simulink model "model_3dof_steering_lateral_selfmade"  (R2022a)
settings: Solver=ode15s  StartTime=0.0  StopTime=para_dura  FixedStep=para_sim_step  MaxStep=para_sim_step  RelTol=1e-9
model workspace (MAT data in the model file):
  SCD_FRESTIMATE_Operating_Point = opcond.OperatingPoint
  SCD_FRESTIMATE_Operating_Point.Model_ = 'model_1dof_longitudinal'
  SCD_FRESTIMATE_Operating_Point.States_(1) = opcond.StatePoint
  SCD_FRESTIMATE_Operating_Point.States_(1).Nx_ = 41
  SCD_FRESTIMATE_Operating_Point.States_(1).Block_ = 'model_1dof_longitudinal/Excitation System/Int Operator'
  SCD_FRESTIMATE_Operating_Point.States_(1).StateName_ = 'v'
  SCD_FRESTIMATE_Operating_Point.States_(1).x_ = [2.02683501926e-10; 1.37568821264e-19; 7.14890844399e-22; 1.12455204277e-20; -7.0630005675e-20; -6.95938068614e-20; 2.72721447959e-21; -3.93535312325e-20; -1.14815977745e-19; 3.30570889294e-20; 3.78600196645e-20; 7.21851569254e-20; -1.77555585105e-19; -2.35291525241e-20; 4.41713994739e-20; -2.05900764101e-21; -1.58367864176e-20; 6.35039836383e-20; -1.30347120926e-20; 1.28680290784e-21; 5.17371795703e-20; 6.49899736287e-20; -4.65181773693e-21; 5.74556218522e-21; -3.90326541642e-20; -4.95314223748e-20; -4.80167923753e-19; 9.22449192438e-20; -2.20085792962e-21; -4.30092800651e-20; -3.42774380714e-20; -1.20947897418e-20; -3.0642370533e-20; -6.43164282462e-20; -2.97515387843e-19; -1.68698506591e-20; 2.312266433e-19; -7.84373380068e-21; 1.67577252929e-20; 2.59801809162e-21; -7.43993193604e-23]
  SCD_FRESTIMATE_Operating_Point.States_(2) = opcond.StatePoint
  SCD_FRESTIMATE_Operating_Point.States_(2).Nx_ = 1
  SCD_FRESTIMATE_Operating_Point.States_(2).Block_ = 'model_1dof_longitudinal/Vehicle Body 1DOF Longitudinal/Vehicle Body 1 DOF/Bus Creation/Body Frame/Longitudinal 1DOF/Integrator3'
  SCD_FRESTIMATE_Operating_Point.States_(2).x_ = 7.28555022085e-16
  SCD_FRESTIMATE_Operating_Point.States_(3) = opcond.StatePoint
  SCD_FRESTIMATE_Operating_Point.States_(3).Nx_ = 1
  SCD_FRESTIMATE_Operating_Point.States_(3).Block_ = 'model_1dof_longitudinal/Vehicle Body 1DOF Longitudinal/Vehicle Body 1 DOF/Integrator1'
  SCD_FRESTIMATE_Operating_Point.States_(3).x_ = -8.63730588445e-16
  SCD_FRESTIMATE_Operating_Point.States_(4) = opcond.StatePoint
  SCD_FRESTIMATE_Operating_Point.States_(4).Nx_ = 1
  SCD_FRESTIMATE_Operating_Point.States_(4).Block_ = 'model_1dof_longitudinal/Vehicle Body 1DOF Longitudinal/Vehicle Body 1 DOF/Vehicle/Integrator'
  SCD_FRESTIMATE_Operating_Point.States_(4).x_ = 1.82750662194e-20
values from neighbouring files (symbols this model uses):
  para_mats = paraStruct.Sv    [main_lateral.m]    (also in main_steering_lateral.m)
  para_sim_matu = paraStruct.SimUv    [main_lateral.m]    (also in main_steering_lateral.m)
  para_sim_step = 5e-4/2    (= 0.00025)    [main_lateral.m]    (also in main_steering_lateral.m = 0.005)
  para_vinit = paraStruct.VInit    [main_lateral.m]    (also in main_steering_lateral.m)
  sim_iun = Simulink.Parameter(1)    [main_lateral.m]    (also in main_steering_lateral.m)
  sim_usnr = zeros(para_sim_usize, 1)    [main_lateral.m]    (also in main_steering_lateral.m)
  ut_pwr = genPower(sim_ut, para_sim_usize)    [main_lateral.m]    (also in main_steering_lateral.m)
undefined symbols (not defined in the file or in its folder): AngSft, AngSW, AVelSft, AVelSW, dpsi, dy, fyf, fyr
libraries: simulink x1
settings Model: SimulationMode=accelerator  PacingRate=1.100000  Creator=无垠穹宇  LastModifiedBy=无垠穹宇
settings SolverCC: ZeroCrossAlgorithm=Adaptive  SolverResetMethod=Robust  MinimalZcImpactIntegration=on  EnableFixedStepZeroCrossing=on
settings DataIOCC: SaveOutput=off  SignalLogging=off  DSMLogging=off  SignalLoggingName=yt
settings OptimizationCC: DefaultParameterBehavior=Inlined  GainParamInheritBuiltInType=on  UseFloatMulNetSlope=on  InlineInvariantSignals=on  EnhancedBackFolding=on  PassReuseOutputArgsThreshold=0  EfficientFloat2IntCast=on  SimCompilerOptimization=on  OptimizeBlockOrder=speed  DifferentSizesBufferReuse=on
settings DebuggingCC: ReadBeforeWriteMsg=DisableAll  WriteAfterWriteMsg=DisableAll  WriteAfterReadMsg=DisableAll  IgnoredZcDiagnostic=none  SolverPrmCheckMsg=warning  MultiTaskDSMMsg=none  ParameterTunabilityLossMsg=error  StateNameClashWarn=warning
settings ModelReferenceCC: UpdateModelReferenceTargets=IfOutOfDate
settings SFSimCC: SFSimEcho=off  SimHardwareAcceleration=native
settings RTWCC: Description=Generic Real-Time Target  RetainRTWFile=on  BuildConfiguration=Faster Runs  CheckMdlBeforeBuild=Warning  DLArmComputeVersion=19.05
settings CodeAppCC: ForceParamTrailComments=on  OperatorAnnotations=on
settings GRTTargetCC: MatFileLogging=off  SupportNonFinite=off

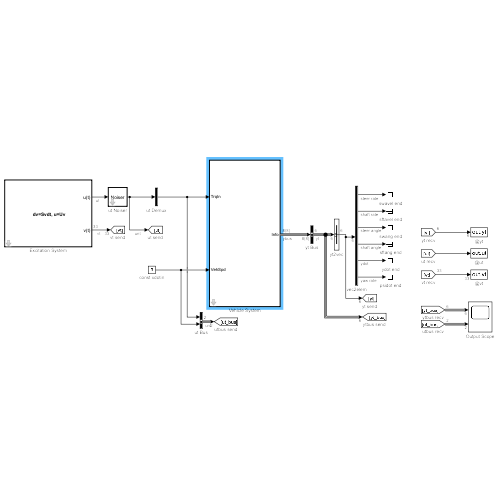
[thumbnail: Simulink's stored preview of the top-level diagram]
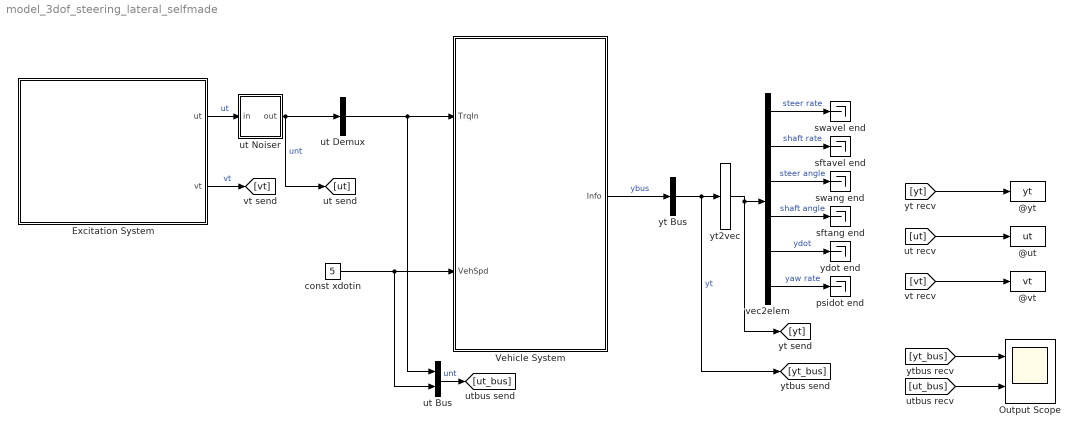
== system model_3dof_steering_lateral_selfmade ==
  @ut : ToWorkspace  VariableName=ut  SaveFormat=Timeseries  SampleTime=para_sim_step
      settings: Decimation=para_resamples
  @vt : ToWorkspace  VariableName=vt  SaveFormat=Timeseries  SampleTime=para_sim_step
      settings: Decimation=para_resamples
  @yt : ToWorkspace  VariableName=yt  SaveFormat=Timeseries  SampleTime=para_sim_step
      settings: Decimation=para_resamples
  Excitation System : Subsystem  TreatAsAtomicUnit=on  mask(State Space with State Vector Output){S=para_mats, U=para_sim_matu, v0=para_vinit}
      mask prompts: S "Matrix S"; U "Matrix U"; v0 "v(0)"
      mask help: 带状态输出的状态空间模型(无控制输入)
      mask DialogControl ParameterGroupVar Prompt: 参数
      mask Display:
      | disp('\bf dv=Svdt, u=Uv', 'texmode', 'on');
      | port_label('output', 1, 'u(t)');
      | port_label('output', 2, 'v(t)');
  Output Scope : Scope  NumInputPorts=2
  Vehicle System : Subsystem  TreatAsAtomicUnit=on  mask(Math Model Parameters){wCf=12e3, wCr=11e3, wIzz=4000, wJ1=0.1, wJ2=0.01, wK=30, wb1=0.001, wb2=1, wb3=0.001, wlf=1.4, wlr=1.6, wm=2000, wxi=0.3, wh=0.35, wTW=1.4, wFznom=5000, wg=9.81}
      mask prompts: wCf "Cf"; wCr "Cr"; wIzz "Izz"; wJ1 "J1"; wJ2 "J2"; wK "K"; wb1 "b1"; wb2 "b2"; wb3 "b3"; wlf "lf"; wlr "lr"; wm "m"; wxi "xi"; wh "h"; wTW "TW"; wFznom "Fznom"; wg "g"
      mask help: 输入状态方程参数, 国际单位制
      settings: MinAlgLoopOccurrences=on
      mask DialogControl ParameterGroupVar Prompt: 参数
  const xdotin : Constant  Value=5  VectorParams1D=off  OutDataTypeStr=double
  psidot end : Terminator
  sftang end : Terminator
  sftavel end : Terminator
  swang end : Terminator
  swavel end : Terminator
  ut Bus : BusCreator  Inputs=2
  ut Demux : Demux  Outputs=1
  ut Noiser : Subsystem  TreatAsAtomicUnit=on  mask(Vectorized AWGN){pwr=ut_pwr, snr=sim_usnr, fmax=20*para_sim_step, judge_para=sim_iun}
      mask prompts: pwr "信号功率向量 (W)"; snr "信噪比向量   (dB)"; fmax "最大动态频率 (1/rad)"; judge_para "噪声启用判断"
      mask help: 给定信号功率和信噪比, 添加高斯白噪声到信号中
      mask DialogControl ParameterGroupVar Prompt: 参数
      mask Display: disp('Noiser');
  vec2elem : Demux  Outputs=6
  ydot end : Terminator
  yt Bus : BusSelector  OutputSignals=shaft info.AVelSW,shaft info.AVelSft,shaft info.AngSW,shaft info.AngSft,body info.dy,body info.dpsi  OutputAsBus=on
  yt2vec : BusToVector
  wires:
  ut Bus/1 -> [ut_bus]  "unt"
  const xdotin/1 -> ut Bus/2, Vehicle System/2(VehSpd)
  ut Noiser/1(out) -> [ut], ut Demux/1  "unt"
  Excitation System/2(vt) -> [vt]  "vt"
  Excitation System/1(ut) -> ut Noiser/1(in)  "ut"
  vec2elem/6 -> psidot end/1  "yaw rate"
  vec2elem/4 -> sftang end/1  "shaft angle"
  vec2elem/5 -> ydot end/1  "ydot"
  yt2vec/1 -> [yt], vec2elem/1
  [yt] -> @yt/1
  vec2elem/3 -> swang end/1  "steer angle"
  [ut] -> @ut/1
  [ut_bus] -> Output Scope/2
  [yt_bus] -> Output Scope/1
  yt Bus/1 -> yt2vec/1, [yt_bus]  "yt"
  [vt] -> @vt/1
  vec2elem/2 -> sftavel end/1  "shaft rate"
  vec2elem/1 -> swavel end/1  "steer rate"
  Vehicle System/1(Info) -> yt Bus/1  "ybus"
  ut Demux/1 -> ut Bus/1, Vehicle System/1(TrqIn)

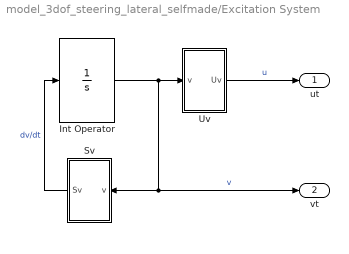
== system model_3dof_steering_lateral_selfmade/Excitation System ==
  Int Operator : Integrator  InitialCondition=v0  WrappedStateUpperValue=1  WrappedStateLowerValue=-1  ContinuousStateAttributes='v'
  Sv : Subsystem
      mask Display: disp('Sv');
  Uv : Subsystem
      mask Display: disp('Uv');
  ut : Outport  OutDataTypeStr=double
  vt : Outport  Port=2  OutDataTypeStr=double
  wires:
  Uv/1(Uv) -> ut/1  "u"
  Int Operator/1 -> Uv/1(v), vt/1, Sv/1(v)  "v"
  Sv/1(Sv) -> Int Operator/1  "dv/dt"

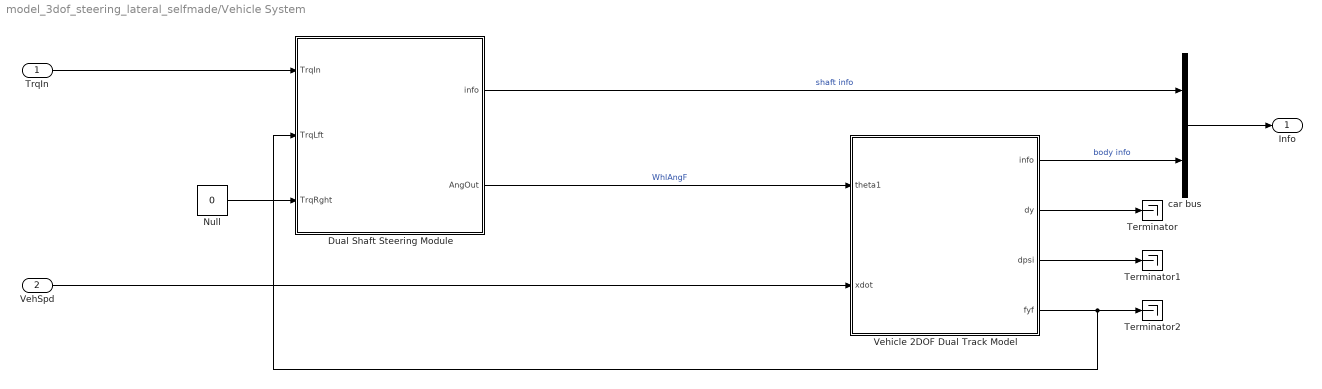
== system model_3dof_steering_lateral_selfmade/Vehicle System ==
  TrqIn : Inport
  VehSpd : Inport  Port=2
  Dual Shaft Steering Module : Subsystem  mask(Dual Shaft Dynamics){J1=wJ1, J2=wJ2, b1=wb1, k1=wK, b2=wb2, b3=wb3, theta_o=0, omega_o=0, xi=wxi, FricTrq=0}
      mask prompts: J1 "vdynblks:vehdynDynamicSteering:blkPrm_J1"; J2 "vdynblks:vehdynDynamicSteering:blkPrm_J2"; b1 "vdynblks:vehdynDynamicSteering:blkPrm_b1"; k1 "vdynblks:vehdynDynamicSteering:blkPrm_k1"; b2 "vdynblks:vehdynDynamicSteering:blkPrm_b3"; b3 "vdynblks:vehdynDynamicSteering:blkPrm_b2"; theta_o "vdynblks:vehdynDynamicSteering:blkPrm_theta_o"; omega_o "vdynblks:vehdynDynamicSteering:blkPrm_omega_o"; xi "trail + pneumatic trail (m)"; FricTrq "vdynblks:vehdynDynamicSteering:blkPrm_FricTrq"
      mask help: 见说明文档
      settings: MinAlgLoopOccurrences=on
      mask Help: eval('vdynblkshelp(''vbsteerdyn'')')
      mask DialogControl J1 Prompt: Steering wheel inertia, J1 [kg*m^2]:
      mask DialogControl J2 Prompt: Steering mechanism inertia, J2 [kg*m^2]:
      mask DialogControl b1 Prompt: Hysteresis viscous damping, b1 [N*m*s/rad]:
      mask DialogControl k1 Prompt: Hysteresis stiffness, k1 [N*m/rad]:
      mask DialogControl b2 Prompt: Steering wheel damping, b2 [N*m*s/rad]:
      mask DialogControl b3 Prompt: Steering mechanism damping, b3 [N*m*s/rad]:
      mask DialogControl theta_o Prompt: Initial steering angle, theta_o [rad]:
      mask DialogControl omega_o Prompt: Initial steering angular velocity, omega_o [rad/s]:
      mask DialogControl FricTrq Prompt: Friction torque, FricTrq [N*m]:
      mask Display:
      | disp('Dual Shaft Dynamics');
      | port_label('input', 1, 'TrqIn');
      | port_label('input', 2, 'TrqLft');
      | port_label('input', 3, 'TrqRght');
      | port_label('output', 1, 'info');
      | port_label('output', 2, 'AngOut');
  Null : Constant  Value=0
  Terminator : Terminator
  Terminator1 : Terminator
  Terminator2 : Terminator
  Vehicle 2DOF Dual Track Model : Subsystem  mask(Vehicle Body 3DOF Lateral){m=wm, h=wh, a=wlf, b=wlr, w=wTW, Cy_f=wCf, Cy_r=wCr, Izz=wIzz, Fznom=wm*wg, g=wg}
      mask prompts: m "autoblks_shared:autoblkVehBody3DofLat:blkPrm_m"; h "Vertical distance from center of mass to axle plane, h [m]:"; a "autoblks_shared:autoblkVehBody3DofLat:blkPrm_a"; b "autoblks_shared:autoblkVehBody3DofLat:blkPrm_b"; w "autoblks_shared:autoblkVehBody3DofLat:blkPrm_w"; Cy_f "autoblks_shared:autoblkVehBody3DofLat:blkPrm_Cy_f"; Cy_r "autoblks_shared:autoblkVehBody3DofLat:blkPrm_Cy_r"; Izz "autoblks_shared:autoblkVehBody3DofLat:blkPrm_Izz"; Fznom "autoblks_shared:autoblkVehBody3DofLat:blkPrm_Fznom"; g "Gravitational acceleration, g [m/s^2]:"
      mask help: autoblks_shared:autoblkVehBody3DofLat:blkDesc
      settings: MinAlgLoopOccurrences=on
      mask Help: eval('autosharedhelp(''vb3doflat'')');
      mask DialogControl ParameterGroupVar Prompt: autoblks_shared:autoblkVehBody3DofLat:blkDlg_ParameterGroupVar
      mask DialogControl LongPanel Prompt: autoblks_shared:autoblkVehBody3DofLat:blkDlg_LongPanel
      mask DialogControl m Prompt: Vehicle mass, m [kg]:
      mask DialogControl a Prompt: Longitudinal distance from center of mass to front axle, a [m]:
      mask DialogControl b Prompt: Longitudinal distance from center of mass to rear axle, b [m]:
      mask DialogControl LatPanel Prompt: autoblks_shared:autoblkVehBody3DofLat:blkDlg_LatPanel
      mask DialogControl w Prompt: Track width, w [m]:
      mask DialogControl Cy_f Prompt: Front tire corner stiffness, Cy_f [N/rad]:
      mask DialogControl Cy_r Prompt: Rear tire axle corner stiffness, Cy_r [N/rad]:
      mask DialogControl YawPanel Prompt: autoblks_shared:autoblkVehBody3DofLat:blkDlg_YawPanel
      mask DialogControl Izz Prompt: Yaw polar inertia, Izz [kg*m^2]:
      mask DialogControl SimPanel Prompt: autoblks_shared:autoblkVehBody3DofLat:blkDlg_SimPanel
      mask DialogControl Fznom Prompt: Nominal normal force, Fznom [N]:
      mask Display:
      | disp('Vehicle 2DOF');
      | port_label('input', 1, 'theta');
      | port_label('input', 2, 'xdot');
      | port_label('output', 1, 'info');
      | port_label('output', 2, 'dy');
      | port_label('output', 3, 'dpsi');
      | port_label('output', 4, 'fyf');
  car bus : BusCreator  Inputs=shaft info,body info
  Info : Outport
  wires:
  Vehicle 2DOF Dual Track Model/1(info) -> car bus/2  "body info"
  car bus/1 -> Info/1
  Null/1 -> Dual Shaft Steering Module/3(TrqRght)
  TrqIn/1 -> Dual Shaft Steering Module/1(TrqIn)
  Dual Shaft Steering Module/1(info) -> car bus/1  "shaft info"
  Vehicle 2DOF Dual Track Model/2(dy) -> Terminator/1
  Vehicle 2DOF Dual Track Model/3(dpsi) -> Terminator1/1
  Vehicle 2DOF Dual Track Model/4(fyf) -> Dual Shaft Steering Module/2(TrqLft), Terminator2/1
  Dual Shaft Steering Module/2(AngOut) -> Vehicle 2DOF Dual Track Model/1(theta1)  "WhlAngF"
  VehSpd/1 -> Vehicle 2DOF Dual Track Model/2(xdot)

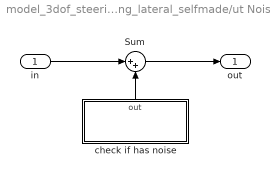
== system model_3dof_steering_lateral_selfmade/ut Noiser ==
  in : Inport  OutDataTypeStr=double
  Sum : Sum  Inputs=|++  AccumDataTypeStr=double  OutDataTypeStr=double
  check if has noise : Subsystem  Variant=on
      mask Display: disp('Variant: awgn/zeros');
  out : Outport  OutDataTypeStr=double
  wires:
  in/1 -> Sum/1
  Sum/1 -> out/1
  check if has noise/1(out) -> Sum/2

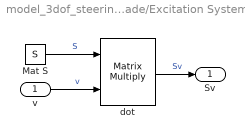
== system model_3dof_steering_lateral_selfmade/Excitation System/Sv ==
  v : Inport  OutDataTypeStr=double
  Mat S : Constant  Value=S  VectorParams1D=off  OutDataTypeStr=double
  dot : Product  Multiplication=Matrix(*)  InputSameDT=on  OutDataTypeStr=double
  Sv : Outport  OutDataTypeStr=double
  wires:
  dot/1 -> Sv/1  "Sv"
  v/1 -> dot/2  "v"
  Mat S/1 -> dot/1  "S"

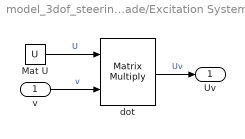
== system model_3dof_steering_lateral_selfmade/Excitation System/Uv ==
  v : Inport  OutDataTypeStr=double
  Mat U : Constant  Value=U  VectorParams1D=off  OutDataTypeStr=double
  dot : Product  Multiplication=Matrix(*)  InputSameDT=on  OutDataTypeStr=double
  Uv : Outport  OutDataTypeStr=double
  wires:
  dot/1 -> Uv/1  "Uv"
  Mat U/1 -> dot/1  "U"
  v/1 -> dot/2  "v"

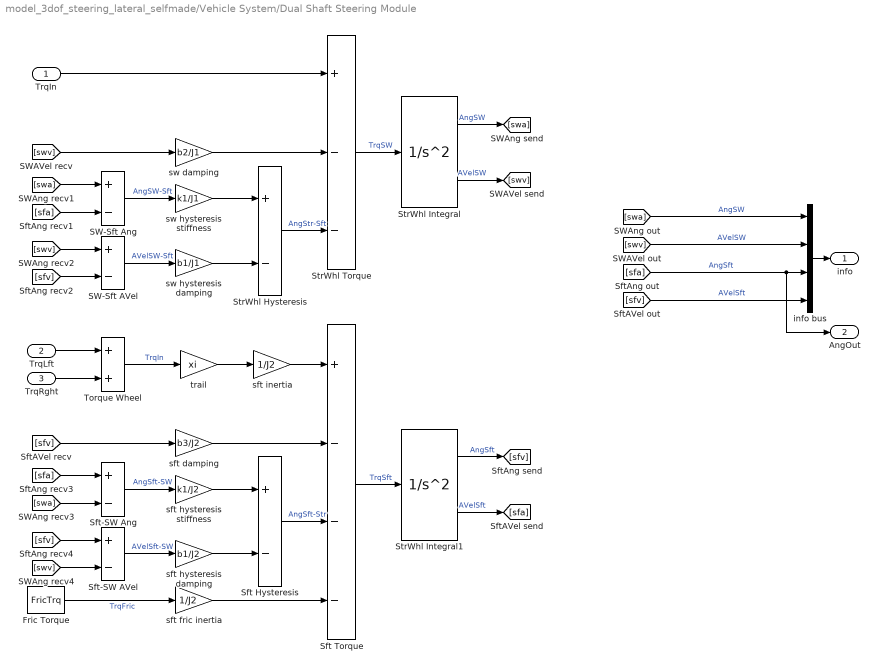
== system model_3dof_steering_lateral_selfmade/Vehicle System/Dual Shaft Steering Module ==
  TrqIn : Inport
  TrqLft : Inport  Port=2
  TrqRght : Inport  Port=3
  Fric Torque : Constant  Value=FricTrq  OutDataTypeStr=double
  SW-Sft AVel : Sum  Inputs=+-  AccumDataTypeStr=double  OutDataTypeStr=double
  SW-Sft Ang : Sum  Inputs=+-  AccumDataTypeStr=double  OutDataTypeStr=double
  Sft Hysteresis : Sum  Inputs=+-  AccumDataTypeStr=double  OutDataTypeStr=double
  Sft Torque : Sum  Inputs=+---  AccumDataTypeStr=double  OutDataTypeStr=double
  Sft-SW AVel : Sum  Inputs=+-  AccumDataTypeStr=double  OutDataTypeStr=double
  Sft-SW Ang : Sum  Inputs=+-  AccumDataTypeStr=double  OutDataTypeStr=double
  StrWhl Hysteresis : Sum  Inputs=+-  AccumDataTypeStr=double  OutDataTypeStr=double
  StrWhl Integral : SecondOrderIntegrator  ICX=theta_o  StateNameX='AngSW'  ICDXDT=omega_o  StateNameDXDT='AVelSW'  IgnoreStateLimitsAndResetForLinearization=on
  StrWhl Integral1 : SecondOrderIntegrator  ICX=theta_o  StateNameX='AngSft'  ICDXDT=omega_o  StateNameDXDT='AVelSft'  IgnoreStateLimitsAndResetForLinearization=on
  StrWhl Torque : Sum  Inputs=+--  AccumDataTypeStr=double  OutDataTypeStr=double
  Torque Wheel : Sum  AccumDataTypeStr=double  OutDataTypeStr=double
  info bus : BusCreator  Inputs=AngSW,AVelSW,AngSft,AVelSft
  sft damping : Gain  Gain=b3/J2  ParamDataTypeStr=double  OutDataTypeStr=double
  sft fric inertia : Gain  Gain=1/J2  ParamDataTypeStr=double  OutDataTypeStr=double
  sft hysteresis damping : Gain  Gain=b1/J2  ParamDataTypeStr=double  OutDataTypeStr=double
  sft hysteresis stiffness : Gain  Gain=k1/J2  ParamDataTypeStr=double  OutDataTypeStr=double
  sft inertia : Gain  Gain=1/J2  ParamDataTypeStr=double  OutDataTypeStr=double
  sw damping : Gain  Gain=b2/J1  ParamDataTypeStr=double  OutDataTypeStr=double
  sw hysteresis damping : Gain  Gain=b1/J1  ParamDataTypeStr=double  OutDataTypeStr=double
  sw hysteresis stiffness : Gain  Gain=k1/J1  ParamDataTypeStr=double  OutDataTypeStr=double
  trail : Gain  Gain=xi  ParamDataTypeStr=double  OutDataTypeStr=double
  info : Outport
  AngOut : Outport  Port=2
  wires:
  StrWhl Torque/1 -> StrWhl Integral/1  "TrqSW"
  sw damping/1 -> StrWhl Torque/2
  sw hysteresis stiffness/1 -> StrWhl Hysteresis/1
  SW-Sft Ang/1 -> sw hysteresis stiffness/1  "AngSW-Sft"
  StrWhl Integral/1 -> [swa]  "AngSW"
  StrWhl Integral/2 -> [swv]  "AVelSW"
  [swa] -> SW-Sft Ang/1
  [swv] -> sw damping/1
  [sfa] -> SW-Sft Ang/2
  TrqIn/1 -> StrWhl Torque/1
  [sfa] -> info bus/3, AngOut/1  "AngSft"
  info bus/1 -> info/1
  [sfv] -> info bus/4  "AVelSft"
  [swa] -> info bus/1  "AngSW"
  [swv] -> info bus/2  "AVelSW"
  StrWhl Hysteresis/1 -> StrWhl Torque/3  "AngStr-Sft"
  [sfv] -> SW-Sft AVel/2
  SW-Sft AVel/1 -> sw hysteresis damping/1  "AVelSW-Sft"
  [swv] -> SW-Sft AVel/1
  sw hysteresis damping/1 -> StrWhl Hysteresis/2
  Sft Hysteresis/1 -> Sft Torque/3  "AngSft-Str"
  sft hysteresis stiffness/1 -> Sft Hysteresis/1
  Sft-SW Ang/1 -> sft hysteresis stiffness/1  "AngSft-SW"
  sft hysteresis damping/1 -> Sft Hysteresis/2
  sft damping/1 -> Sft Torque/2
  StrWhl Integral1/1 -> [sfv]  "AngSft"
  Sft Torque/1 -> StrWhl Integral1/1  "TrqSft"
  StrWhl Integral1/2 -> [sfa]  "AVelSft"
  Sft-SW AVel/1 -> sft hysteresis damping/1  "AVelSft-SW"
  [sfv] -> sft damping/1
  Torque Wheel/1 -> trail/1  "TrqIn"
  TrqLft/1 -> Torque Wheel/1
  TrqRght/1 -> Torque Wheel/2
  sft inertia/1 -> Sft Torque/1
  Fric Torque/1 -> sft fric inertia/1  "TrqFric"
  sft fric inertia/1 -> Sft Torque/4
  [swa] -> Sft-SW Ang/2
  [sfa] -> Sft-SW Ang/1
  [sfv] -> Sft-SW AVel/1
  [swv] -> Sft-SW AVel/2
  trail/1 -> sft inertia/1

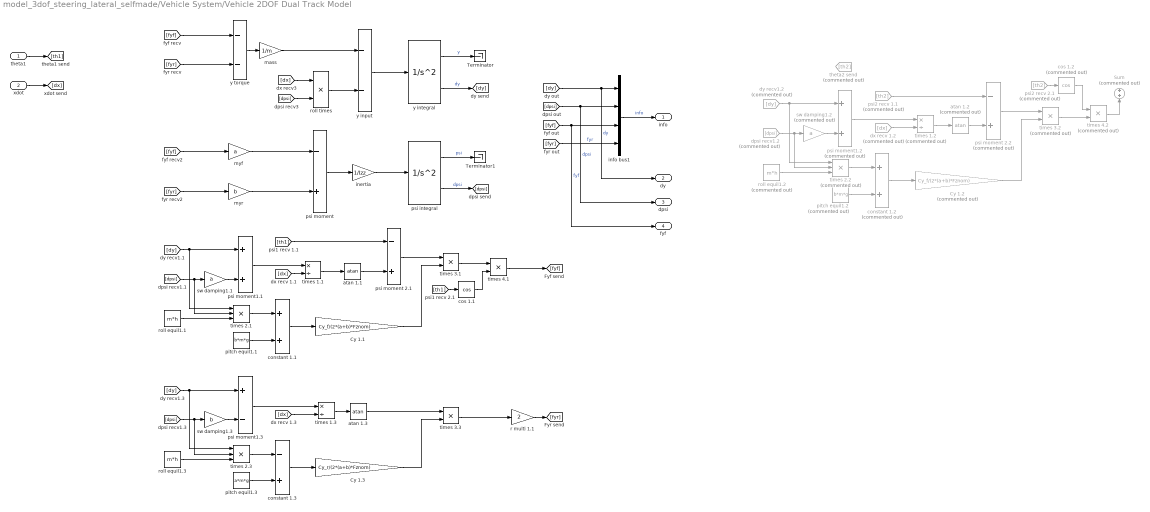
== system model_3dof_steering_lateral_selfmade/Vehicle System/Vehicle 2DOF Dual Track Model ==
  theta1 : Inport
  xdot : Inport  Port=2
  Cy 1.1 : Gain  Gain=Cy_f/(2*(a+b)*Fznom)  ParamDataTypeStr=double  OutDataTypeStr=double
  Cy 1.2 : Gain  Commented=on  Gain=Cy_f/(2*(a+b)*Fznom)  ParamDataTypeStr=double  OutDataTypeStr=double
  Cy 1.3 : Gain  Gain=Cy_r/(2*(a+b)*Fznom)  ParamDataTypeStr=double  OutDataTypeStr=double
  Sum : Sum  Commented=on  Inputs=+|+  AccumDataTypeStr=double  OutDataTypeStr=double
  Terminator : Terminator
  Terminator1 : Terminator
  atan 1.1 : Trigonometry  Operator=atan  OutputSignalType=real
  atan 1.2 : Trigonometry  Commented=on  Operator=atan  OutputSignalType=real
  atan 1.3 : Trigonometry  Operator=atan  OutputSignalType=real
  constant 1.1 : Sum  AccumDataTypeStr=double  OutDataTypeStr=double
  constant 1.2 : Sum  Commented=on  AccumDataTypeStr=double  OutDataTypeStr=double
  constant 1.3 : Sum  Inputs=-+  AccumDataTypeStr=double  OutDataTypeStr=double
  cos 1.1 : Trigonometry  Operator=cos  OutputSignalType=real
  cos 1.2 : Trigonometry  Commented=on  Operator=cos  OutputSignalType=real
  dpsi recv1.2 : From  Commented=on  GotoTag=dpsi
  dx recv 1.2 : From  Commented=on  GotoTag=dx
  dy recv1.2 : From  Commented=on  GotoTag=dy
  inertia : Gain  Gain=1/Izz  ParamDataTypeStr=double  OutDataTypeStr=double
  info bus1 : BusCreator  Inputs=dy,dpsi,fyf,fyr
  mass : Gain  Gain=1/m  ParamDataTypeStr=double  OutDataTypeStr=double
  myf : Gain  Gain=a  ParamDataTypeStr=double  OutDataTypeStr=double
  myr : Gain  Gain=b  ParamDataTypeStr=double  OutDataTypeStr=double
  pitch equil1.1 : Constant  Value=b*m*g  OutDataTypeStr=double
  pitch equil1.2 : Constant  Commented=on  Value=b*m*g  OutDataTypeStr=double
  pitch equil1.3 : Constant  Value=a*m*g  OutDataTypeStr=double
  psi integral : SecondOrderIntegrator  ICX=0  StateNameX='psi_ang'  ICDXDT=0  StateNameDXDT='psi_avel'  IgnoreStateLimitsAndResetForLinearization=on
  psi moment : Sum  Inputs=-+  AccumDataTypeStr=double  OutDataTypeStr=double
  psi moment 2.1 : Sum  Inputs=-+  AccumDataTypeStr=double  OutDataTypeStr=double
  psi moment 2.2 : Sum  Commented=on  Inputs=-+  AccumDataTypeStr=double  OutDataTypeStr=double
  psi moment1.1 : Sum  AccumDataTypeStr=double  OutDataTypeStr=double
  psi moment1.2 : Sum  Commented=on  AccumDataTypeStr=double  OutDataTypeStr=double
  psi moment1.3 : Sum  Inputs=+-  AccumDataTypeStr=double  OutDataTypeStr=double
  psi2 recv 1.1 : From  Commented=on  GotoTag=th2
  psi2 recv 2.1 : From  Commented=on  GotoTag=th2
  r multi 1.1 : Gain  Gain=2  ParamDataTypeStr=double  OutDataTypeStr=double
  roll equil1.1 : Constant  Value=m*h  OutDataTypeStr=double
  roll equil1.2 : Constant  Commented=on  Value=m*h  OutDataTypeStr=double
  roll equil1.3 : Constant  Value=m*h  OutDataTypeStr=double
  roll times : Product  Inputs=**
  sw damping1.1 : Gain  Gain=a  ParamDataTypeStr=double  OutDataTypeStr=double
  sw damping1.2 : Gain  Commented=on  Gain=a  ParamDataTypeStr=double  OutDataTypeStr=double
  sw damping1.3 : Gain  Gain=b  ParamDataTypeStr=double  OutDataTypeStr=double
  theta2 send : Goto  Commented=on  GotoTag=th2
  times 1.1 : Product  Inputs=*/
  times 1.2 : Product  Commented=on  Inputs=*/
  times 1.3 : Product  Inputs=*/
  times 2.1 : Product  Inputs=***  OutDataTypeStr=double
  times 2.2 : Product  Commented=on  Inputs=***  OutDataTypeStr=double
  times 2.3 : Product  Inputs=***  OutDataTypeStr=double
  times 3.1 : Product  Inputs=**  OutDataTypeStr=double
  times 3.2 : Product  Commented=on  Inputs=**  OutDataTypeStr=double
  times 3.3 : Product  Inputs=**  OutDataTypeStr=double
  times 4.1 : Product  Inputs=**  OutDataTypeStr=double
  times 4.2 : Product  Commented=on  Inputs=**  OutDataTypeStr=double
  y input : Sum  Inputs=--  AccumDataTypeStr=double  OutDataTypeStr=double
  y integral : SecondOrderIntegrator  ICX=0  StateNameX='y'  ICDXDT=0  StateNameDXDT='dy'  IgnoreStateLimitsAndResetForLinearization=on
  y torque : Sum  Inputs=--  AccumDataTypeStr=double  OutDataTypeStr=double
  info : Outport
  dy : Outport  Port=2
  dpsi : Outport  Port=3
  fyf : Outport  Port=4
  wires:
  y torque/1 -> mass/1
  theta1/1 -> [th1]
  xdot/1 -> [dx]
  y integral/1 -> Terminator/1  "y"
  y integral/2 -> [dy]  "dy"
  psi integral/1 -> Terminator1/1  "psi"
  psi integral/2 -> [dpsi]  "dpsi"
  [dy] -> times 2.1/1, psi moment1.1/1
  sw damping1.1/1 -> psi moment1.1/2
  psi moment1.1/1 -> times 1.1/1
  [dx] -> times 1.1/2
  [th1] -> psi moment 2.1/1
  [dpsi] -> times 2.1/2, sw damping1.1/1
  mass/1 -> y input/1
  y input/1 -> y integral/1
  [dx] -> roll times/1
  [dpsi] -> roll times/2
  roll times/1 -> y input/2
  psi moment/1 -> inertia/1
  [fyf] -> myf/1
  [fyr] -> myr/1
  inertia/1 -> psi integral/1
  [dy] -> dy/1, info bus1/1  "dy"
  [dpsi] -> dpsi/1, info bus1/2  "dpsi"
  [fyf] -> fyf/1, info bus1/3  "fyf"
  [fyr] -> info bus1/4  "fyr"
  info bus1/1 -> info/1  "info"
  r multi 1.1/1 -> [fyr]
  [fyf] -> y torque/1
  [fyr] -> y torque/2
  myf/1 -> psi moment/1
  myr/1 -> psi moment/2
  times 4.1/1 -> [fyf]
  roll equil1.1/1 -> times 2.1/3
  pitch equil1.1/1 -> constant 1.1/2
  times 2.1/1 -> constant 1.1/1
  constant 1.1/1 -> Cy 1.1/1
  psi moment 2.1/1 -> times 3.1/1
  Cy 1.1/1 -> times 3.1/2
  Cy 1.2/1 -> times 3.2/2
  times 2.2/1 -> constant 1.2/1
  roll equil1.2/1 -> times 2.2/3
  constant 1.2/1 -> Cy 1.2/1
  pitch equil1.2/1 -> constant 1.2/2
  dpsi recv1.2/1 -> times 2.2/2, sw damping1.2/1
  sw damping1.2/1 -> psi moment1.2/2
  psi2 recv 1.1/1 -> psi moment 2.2/1
  dy recv1.2/1 -> times 2.2/1, psi moment1.2/1
  psi moment1.2/1 -> times 1.2/1
  dx recv 1.2/1 -> times 1.2/2
  psi moment 2.2/1 -> times 3.2/1
  [dy] -> times 2.3/1, psi moment1.3/1
  [dpsi] -> times 2.3/2, sw damping1.3/1
  sw damping1.3/1 -> psi moment1.3/2
  times 1.3/1 -> atan 1.3/1
  psi moment1.3/1 -> times 1.3/1
  pitch equil1.3/1 -> constant 1.3/2
  constant 1.3/1 -> Cy 1.3/1
  times 2.3/1 -> constant 1.3/1
  Cy 1.3/1 -> times 3.3/2
  roll equil1.3/1 -> times 2.3/3
  [dx] -> times 1.3/2
  times 3.3/1 -> r multi 1.1/1
  times 3.1/1 -> times 4.1/1
  times 3.2/1 -> times 4.2/2
  [th1] -> cos 1.1/1
  cos 1.1/1 -> times 4.1/2
  psi2 recv 2.1/1 -> cos 1.2/1
  cos 1.2/1 -> times 4.2/1
  times 1.1/1 -> atan 1.1/1
  atan 1.1/1 -> psi moment 2.1/2
  times 1.2/1 -> atan 1.2/1
  atan 1.2/1 -> psi moment 2.2/2
  atan 1.3/1 -> times 3.3/1
  times 4.2/1 -> Sum/2

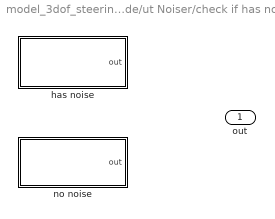
== system model_3dof_steering_lateral_selfmade/ut Noiser/check if has noise ==
  has noise : Subsystem  TreatAsAtomicUnit=on  VariantControl=judge_para == 0
  no noise : Subsystem  TreatAsAtomicUnit=on  VariantControl=judge_para ~= 0
  out : Outport  OutDataTypeStr=double

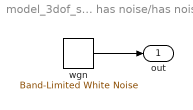
== system model_3dof_steering_lateral_selfmade/ut Noiser/check if has noise/has noise ==
  wgn : simulink/Sources/Band-Limited White Noise  Cov=pwr./(10.^(snr./10)).*(2*pi/(100*fmax))  Ts=2*pi/(100*fmax)  seed=[23341]
  out : Outport  OutDataTypeStr=double
  wires:
  wgn/1 -> out/1

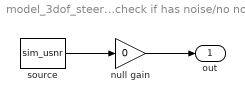
== system model_3dof_steering_lateral_selfmade/ut Noiser/check if has noise/no noise ==
  null gain : Gain  Gain=0  ParamDataTypeStr=double  OutDataTypeStr=double
  source : Constant  Value=sim_usnr  OutDataTypeStr=double
  out : Outport
  wires:
  null gain/1 -> out/1
  source/1 -> null gain/1
